simulink model "std_opsaet"  (R2016a)
settings: Solver=VariableStepAuto  StartTime=0.0  StopTime=10.0  RelTol=1e-3
settings Model: Creator=henri  LastModifiedBy=henri

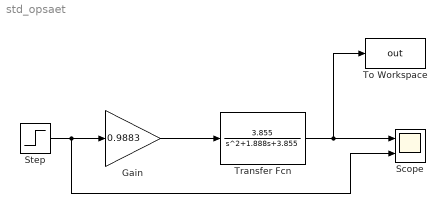
== system std_opsaet ==
  Gain : Gain  Gain=0.9883
  Scope : Scope  NumInputPorts=2
  Step : Step  Time=0.5  Before=1.56  After=2.46  SampleTime=0
  To Workspace : ToWorkspace  VariableName=out  SaveFormat=Timeseries  SampleTime=-1
  Transfer Fcn : TransferFcn  Numerator=[3.855]  Denominator=[1 1.888 3.855]
  wires:
  Gain/1 -> Transfer Fcn/1
  Transfer Fcn/1 -> To Workspace/1, Scope/1
  Step/1 -> Scope/2, Gain/1
